simulink model "motor_SMC"  (R2016b)
settings: Solver=VariableStepAuto  StartTime=0.0  StopTime=10  RelTol=1e-3
settings Model: Creator=lqy  LastModifiedBy=96919
settings DataIOCC: ReturnWorkspaceOutputs=on  ReturnWorkspaceOutputsName=spidata

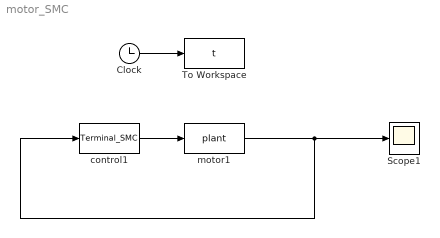
== system motor_SMC ==
  Clock : Clock
  Scope1 : Scope
  To Workspace : ToWorkspace  VariableName=t  SampleTime=-1
  control1 : S-Function  FunctionName=Terminal_SMC  SFunctionDeploymentMode=off  EnableBusSupport=off
  motor1 : S-Function  FunctionName=plant  SFunctionDeploymentMode=off  EnableBusSupport=off
  wires:
  Clock/1 -> To Workspace/1
  motor1/1 -> control1/1, Scope1/1
  control1/1 -> motor1/1
